simulink model "ejercicio_5"  (R2020b)
settings: Solver=ode4  StartTime=0.0  StopTime=30.0  FixedStep=0.05  MaxStep=0.01  RelTol=1e-3
settings Model: EnablePacing=on  Creator=alexa  LastModifiedBy=alexa

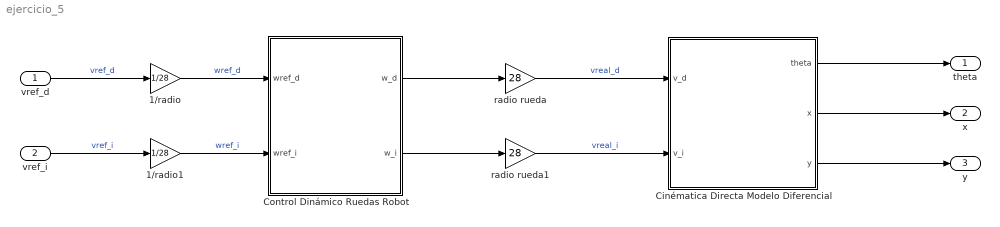
== system ejercicio_5 ==
  vref_d : Inport
  vref_i : Inport  Port=2
  1/radio : Gain  Gain=1/28
  1/radio1 : Gain  Gain=1/28
  Cinématica Directa Modelo Diferencial : Subsystem  mask{b=56}
      mask prompts: b "Distancia entre ruedas:"
  Control Dinámico Ruedas Robot : Subsystem
  radio rueda : Gain  Gain=28
  radio rueda1 : Gain  Gain=28
  theta : Outport
  x : Outport  Port=2
  y : Outport  Port=3
  wires:
  vref_d/1 -> 1/radio/1  "vref_d"
  vref_i/1 -> 1/radio1/1  "vref_i"
  radio rueda/1 -> Cinématica Directa Modelo Diferencial/1(v_d)  "vreal_d"
  radio rueda1/1 -> Cinématica Directa Modelo Diferencial/2(v_i)  "vreal_i"
  1/radio/1 -> Control Dinámico Ruedas Robot/1(wref_d)  "wref_d"
  1/radio1/1 -> Control Dinámico Ruedas Robot/2(wref_i)  "wref_i"
  Control Dinámico Ruedas Robot/1(w_d) -> radio rueda/1
  Control Dinámico Ruedas Robot/2(w_i) -> radio rueda1/1
  Cinématica Directa Modelo Diferencial/1(theta) -> theta/1
  Cinématica Directa Modelo Diferencial/2(x) -> x/1
  Cinématica Directa Modelo Diferencial/3(y) -> y/1

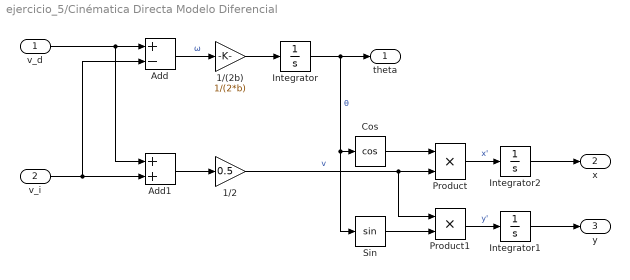
== system ejercicio_5/Cinématica Directa Modelo Diferencial ==
  v_d : Inport
  v_i : Inport  Port=2
  1/(2b) : Gain  Gain=1/(2*b)
  1/2 : Gain  Gain=0.5
  Add : Sum  Inputs=+-
  Add1 : Sum
  Cos : Trigonometry  Operator=cos
  Integrator : Integrator
  Integrator1 : Integrator
  Integrator2 : Integrator
  Product : Product
  Product1 : Product
  Sin : Trigonometry
  theta : Outport
  x : Outport  Port=2
  y : Outport  Port=3
  wires:
  Cos/1 -> Product/1
  Add/1 -> 1/(2b)/1  "ω"
  Product/1 -> Integrator2/1  "x'"
  1/2/1 -> Product1/1, Product/2  "v"
  Product1/1 -> Integrator1/1  "y'"
  Sin/1 -> Product1/2
  Integrator1/1 -> y/1
  Integrator/1 -> theta/1, Sin/1, Cos/1  "θ"
  v_i/1 -> Add/2, Add1/2
  v_d/1 -> Add1/1, Add/1
  Add1/1 -> 1/2/1
  Integrator2/1 -> x/1
  1/(2b)/1 -> Integrator/1

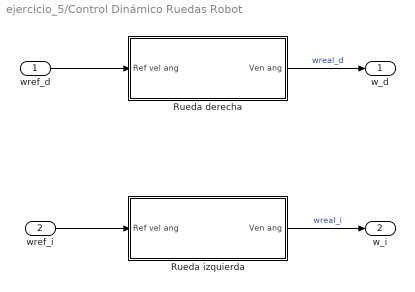
== system ejercicio_5/Control Dinámico Ruedas Robot ==
  wref_d : Inport
  wref_i : Inport  Port=2
  Rueda derecha : Subsystem  mask{tau=0.09, kp=3, k=0.2}
      mask prompts: tau "Valor cte tiempo motor:"; kp "Valor ganancia regulador P:"; k "Valor ganancia motor:"
  Rueda izquierda : Subsystem  mask{k=3, tau=0.09, kp=0.2}
      mask prompts: k "Valor ganancia motor:"; tau "Valor cte tiempo motor:"; kp "Valor ganancia regulador P:"
  w_d : Outport
  w_i : Outport  Port=2
  wires:
  wref_d/1 -> Rueda derecha/1(Ref vel ang)
  wref_i/1 -> Rueda izquierda/1(Ref vel ang)
  Rueda derecha/1(Ven ang) -> w_d/1  "wreal_d"
  Rueda izquierda/1(Ven ang) -> w_i/1  "wreal_i"

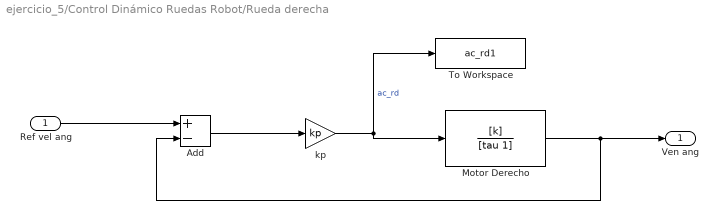
== system ejercicio_5/Control Dinámico Ruedas Robot/Rueda derecha ==
  Ref vel ang : Inport
  Add : Sum  Inputs=+-
  Motor Derecho : TransferFcn  Numerator=[k]  Denominator=[tau 1]
  To Workspace : ToWorkspace  VariableName=ac_rd1  SaveFormat=Timeseries  SampleTime=-1
  kp : Gain  Gain=kp
  Ven ang : Outport
  wires:
  Add/1 -> kp/1
  kp/1 -> To Workspace/1, Motor Derecho/1  "ac_rd"
  Motor Derecho/1 -> Add/2, Ven ang/1
  Ref vel ang/1 -> Add/1

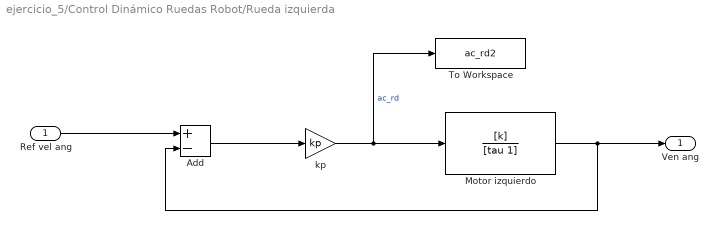
== system ejercicio_5/Control Dinámico Ruedas Robot/Rueda izquierda ==
  Ref vel ang : Inport
  Add : Sum  Inputs=+-
  Motor izquierdo : TransferFcn  Numerator=[k]  Denominator=[tau 1]
  To Workspace : ToWorkspace  VariableName=ac_rd2  SaveFormat=Timeseries  SampleTime=-1
  kp : Gain  Gain=kp
  Ven ang : Outport
  wires:
  Add/1 -> kp/1
  kp/1 -> To Workspace/1, Motor izquierdo/1  "ac_rd"
  Motor izquierdo/1 -> Ven ang/1, Add/2
  Ref vel ang/1 -> Add/1
